simulink model "s9_template_2019a"  (R2019a)
settings: Solver=ode4  StartTime=0.0  StopTime=inf  FixedStep=P_sim_dt  RelTol=1e-3
InitFcn:
  | s6_data;
values from neighbouring files (symbols this model uses):
  init_psi = -pi/2    (= -1.57079632679)    [s6_data.m]
  init_s1 = a1boundary + P_width/2    (= 0.15)    [s6_data.m]
  init_s2 = a2total/2    (= 0.9)    [s6_data.m]
  P_delta_n_max = 1    [s6_data.m]
  P_delta_n_min = -1    [s6_data.m]
  P_dt = 20e-3    (= 0.02)    [s6_data.m]
  P_kr = 1/P_ku * sqrt((P_Ti^2*P_omega_d^2 + P_T^2*P_Ti^2*P_omega_d^4) /     (1 + P_Ti^2*P_omega_d^2))    [ex6_1.m]    (also in s6_data.m = sqrt((P_omega_d^2*P_T*P_Ti)^2 + (P_omega_d*P_Ti)^2) /      ()
  P_Ta = 0.02    [ex6_1.m]    (also in s6_data.m)
  P_Ti = (tan(P_phires_arc - pi + P_Tt*P_omega_d) * P_T * P_omega_d - 1)/     (P_T*P_omega_d^2 + tan(P_phires_arc - pi + P_Tt*P_omega_d) * P_omega_d )    [ex6_1.m]    (also in s6_data.m = tan(P_phi_res - pi/2 + P_omega_d*P_Tt + atan(P_omega_d*P_T)))
  P_Tw = 1000e-3    (= 1)    [ex6_1.m]    (also in s6_data.m = 0.3)
  P_un_max = 1    [s6_data.m]
  P_un_min = -1    [s6_data.m]
  P_v_fb_border = 0.1    [s6_data.m]
  P_vTarget = 0.3    [s6_data.m]
  P_w_breakslen = uint32(length(path.points))    [s6_data.m]
  P_w_coefs = zeros(SPLINE.Elements(3).Dimensions)    [s6_data.m]
  P_w_points = zeros(SPLINE.Elements(2).Dimensions)    [s6_data.m]
  P_w_segments = uint32(zeros(SPLINE.Elements(4).Dimensions))    [s6_data.m]
  track = mbc_track_display(track, 0.1, [ 0 a1total 0 a2total ])    [s6_data.m]
undefined symbols (not defined in the file or in its folder): CarInputsCmdForward, disableLaneMonitor, isnew, lapCount, ManeuverTypePathFollow, P_p_Bf, P_p_Br, P_p_Cf, P_p_Cr, P_p_delta_max, P_p_delta_min, P_p_Df, P_p_Dr, P_p_frontaxle_1, P_p_J, P_p_k, P_p_l, P_p_m, P_p_rearaxle_1, P_p_T, P_p_un_max, P_p_un_min, P_p_un_slow_max, P_p_un_slow_min, P_p_uTt, P_p_v_min, type, vmax, xManeuverEnd
libraries: mad_lib_template x1
settings Model: Creator=hmekiedj  LastModifiedBy=exdestruction
settings DataIOCC: ReturnWorkspaceOutputs=off
settings DebuggingCC: ArithmeticOperatorsInVariantConditions=warning
settings SFSimCC: SimUseLocalCustomCode=off
settings RTWCC: RTWUseLocalCustomCode=off

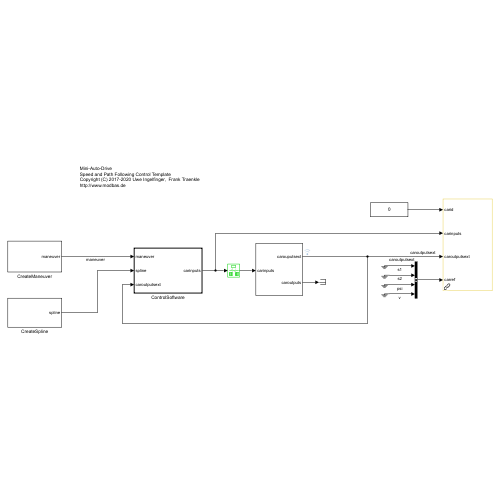
[thumbnail: Simulink's stored preview of the top-level diagram]
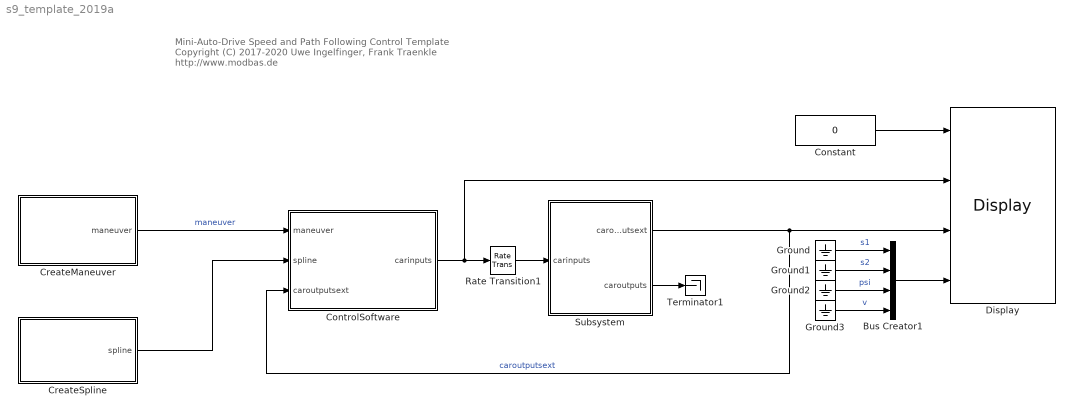
== system s9_template_2019a ==
  note: Mini-Auto-Drive
      | Speed and Path Following Control Template
      | Copyright (C) 2017-2020 Uwe Ingelfinger,  Frank Traenkle
      | http://www.modbas.de
  Bus Creator1 : BusCreator  Inputs=4
  Constant : Constant  Value=0
  ControlSoftware : Subsystem  TreatAsAtomicUnit=on  SystemSampleTime=P_dt
  CreateManeuver : Subsystem
  CreateSpline : Subsystem
  Display : mad_lib_template/Display  SystemSampleTime=-1  Latency=0  AutoFrameSizeCalculation=off
  Ground{,1..3} (4 alike) : Ground
  Rate Transition1 : RateTransition
  Subsystem : Subsystem
  Terminator1 : Terminator
  wires:
  Bus Creator1/1 -> Display/4
  Ground/1 -> Bus Creator1/1  "s1"
  Ground1/1 -> Bus Creator1/2  "s2"
  Ground2/1 -> Bus Creator1/3  "psi"
  Ground3/1 -> Bus Creator1/4  "v"
  Subsystem/1(carouputsext) -> ControlSoftware/3(caroutputsext), Display/3  "caroutputsext"
  Rate Transition1/1 -> Subsystem/1(carinputs)
  Constant/1 -> Display/1
  ControlSoftware/1(carinputs) -> Display/2, Rate Transition1/1
  CreateManeuver/1(maneuver) -> ControlSoftware/1(maneuver)  "maneuver"
  Subsystem/2(caroutputs) -> Terminator1/1
  CreateSpline/1(spline) -> ControlSoftware/2(spline)

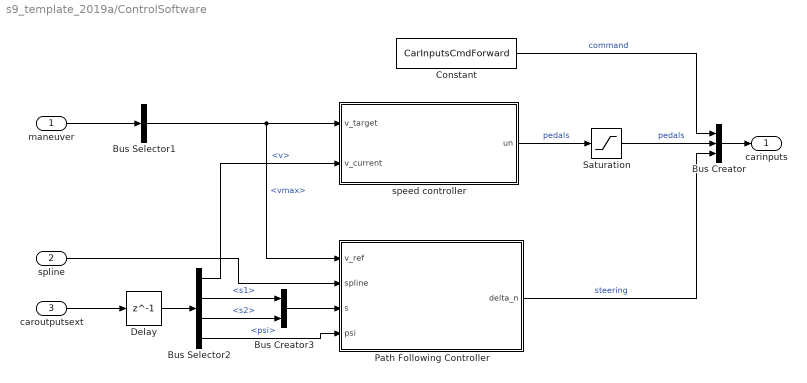
== system s9_template_2019a/ControlSoftware ==
  maneuver : Inport
  spline : Inport  Port=2
  caroutputsext : Inport  Port=3
  Bus Creator : BusCreator  Inputs=3
  Bus Creator3 : BusCreator  Inputs=2
  Bus Selector1 : BusSelector  OutputSignals=vmax
  Bus Selector2 : BusSelector  OutputSignals=v,s1,s2,psi
  Constant : Constant  Value=CarInputsCmdForward  SampleTime=-1
  Delay : Delay  DelayLength=1
  Path Following Controller : Subsystem
  Saturation : Saturate  UpperLimit=P_un_max  LowerLimit=P_un_min
  speed controller : Subsystem  TreatAsAtomicUnit=on  SystemSampleTime=P_dt
      settings: MinAlgLoopOccurrences=on
  carinputs : Outport
  wires:
  caroutputsext/1 -> Delay/1
  Bus Creator/1 -> carinputs/1
  maneuver/1 -> Bus Selector1/1
  speed controller/1(un) -> Saturation/1  "pedals"
  Saturation/1 -> Bus Creator/2  "pedals"
  Constant/1 -> Bus Creator/1  "command"
  Path Following Controller/1(delta_n) -> Bus Creator/3  "steering"
  Bus Creator3/1 -> Path Following Controller/3(s)
  Bus Selector2/1 -> speed controller/2(v_current)  "<v>"
  Bus Selector2/2 -> Bus Creator3/1  "<s1>"
  Bus Selector2/4 -> Path Following Controller/4(psi)  "<psi>"
  Bus Selector2/3 -> Bus Creator3/2  "<s2>"
  Bus Selector1/1 -> Path Following Controller/1(v_ref), speed controller/1(v_target)  "<vmax>"
  Delay/1 -> Bus Selector2/1
  spline/1 -> Path Following Controller/2(spline)

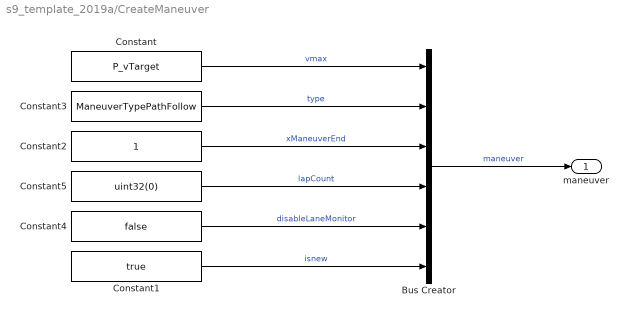
== system s9_template_2019a/CreateManeuver ==
  Bus Creator : BusCreator  Inputs=vmax,type,xManeuverEnd,lapCount,disableLaneMonitor,isnew  OutDataTypeStr=Bus: MANEUVER  NonVirtualBus=on
  Constant : Constant  Value=P_vTarget
  Constant1 : Constant  Value=true
  Constant2 : Constant
  Constant3 : Constant  Value=ManeuverTypePathFollow
  Constant4 : Constant  Value=false
  Constant5 : Constant  Value=uint32(0)
  maneuver : Outport
  wires:
  Bus Creator/1 -> maneuver/1  "maneuver"
  Constant3/1 -> Bus Creator/2  "type"
  Constant2/1 -> Bus Creator/3  "xManeuverEnd"
  Constant4/1 -> Bus Creator/5  "disableLaneMonitor"
  Constant5/1 -> Bus Creator/4  "lapCount"
  Constant1/1 -> Bus Creator/6  "isnew"
  Constant/1 -> Bus Creator/1  "vmax"

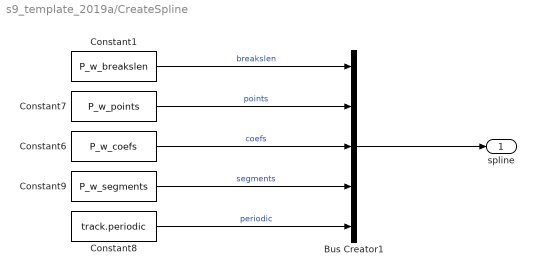
== system s9_template_2019a/CreateSpline ==
  Bus Creator1 : BusCreator  Inputs=5  OutDataTypeStr=Bus: SPLINE  NonVirtualBus=on
  Constant1 : Constant  Value=P_w_breakslen  VectorParams1D=off
  Constant6 : Constant  Value=P_w_coefs  VectorParams1D=off
  Constant7 : Constant  Value=P_w_points  VectorParams1D=off
  Constant8 : Constant  Value=track.periodic  VectorParams1D=off
  Constant9 : Constant  Value=P_w_segments  VectorParams1D=off
  spline : Outport
  wires:
  Constant1/1 -> Bus Creator1/1  "breakslen"
  Constant8/1 -> Bus Creator1/5  "periodic"
  Constant9/1 -> Bus Creator1/4  "segments"
  Constant6/1 -> Bus Creator1/3  "coefs"
  Constant7/1 -> Bus Creator1/2  "points"
  Bus Creator1/1 -> spline/1

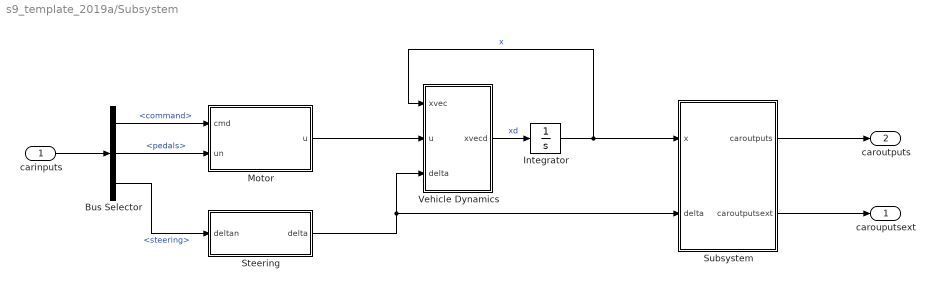
== system s9_template_2019a/Subsystem ==
  carinputs : Inport
  Bus Selector : BusSelector  OutputSignals=command,pedals,steering
  Integrator : Integrator  InitialCondition=[ 0; init_s1; init_s2; init_psi; 0; 0; 0]
  Motor : Subsystem
  Steering : Subsystem
  Subsystem : Subsystem
  Vehicle Dynamics : MATLAB Function  TreatAsAtomicUnit=on
  carouputsext : Outport
  caroutputs : Outport  Port=2
  wires:
  Vehicle Dynamics/1(xvecd) -> Integrator/1  "xd"
  Motor/1(u) -> Vehicle Dynamics/2(u)
  carinputs/1 -> Bus Selector/1
  Integrator/1 -> Subsystem/1(x), Vehicle Dynamics/1(xvec)  "x"
  Bus Selector/3 -> Steering/1(deltan)  "<steering>"
  Steering/1(delta) -> Subsystem/2(delta), Vehicle Dynamics/3(delta)
  Bus Selector/2 -> Motor/2(un)  "<pedals>"
  Bus Selector/1 -> Motor/1(cmd)  "<command>"
  Subsystem/1(caroutputs) -> caroutputs/1
  Subsystem/2(caroutputsext) -> carouputsext/1

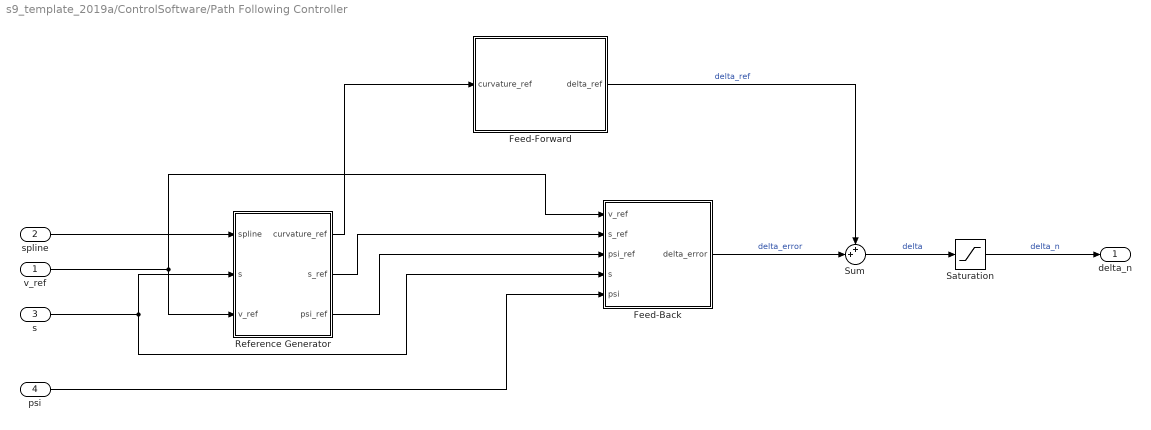
== system s9_template_2019a/ControlSoftware/Path Following Controller ==
  v_ref : Inport
  spline : Inport  Port=2
  s : Inport  Port=3
  psi : Inport  Port=4
  Feed-Back : Subsystem
  Feed-Forward : Subsystem
  Reference Generator : Subsystem
  Saturation : Saturate  UpperLimit=P_delta_n_max  LowerLimit=P_delta_n_min
  Sum : Sum  Inputs=++|
  delta_n : Outport
  wires:
  Saturation/1 -> delta_n/1  "delta_n"
  Sum/1 -> Saturation/1  "delta"
  Feed-Back/1(delta_error) -> Sum/2  "delta_error"
  Reference Generator/2(s_ref) -> Feed-Back/2(s_ref)
  Reference Generator/3(psi_ref) -> Feed-Back/3(psi_ref)
  s/1 -> Feed-Back/4(s), Reference Generator/2(s)
  psi/1 -> Feed-Back/5(psi)
  Reference Generator/1(curvature_ref) -> Feed-Forward/1(curvature_ref)
  v_ref/1 -> Feed-Back/1(v_ref), Reference Generator/3(v_ref)
  Feed-Forward/1(delta_ref) -> Sum/1  "delta_ref"
  spline/1 -> Reference Generator/1(spline)

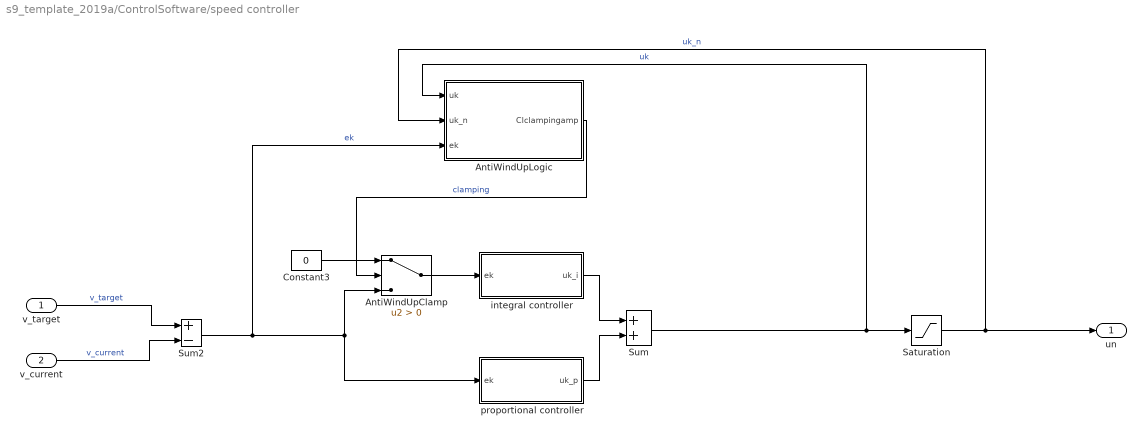
== system s9_template_2019a/ControlSoftware/speed controller ==
  v_target : Inport
  v_current : Inport  Port=2
  AntiWindUpClamp : Switch  Criteria=u2 > Threshold
  AntiWindUpLogic : Subsystem
  Constant3 : Constant  Value=0
  Saturation : Saturate  UpperLimit=P_un_max  LowerLimit=P_un_min
  Sum : Sum
  Sum2 : Sum  Inputs=+-
  integral controller : Subsystem
  proportional controller : Subsystem
  un : Outport
  wires:
  Saturation/1 -> AntiWindUpLogic/2(uk_n), un/1  "uk_n"
  Sum2/1 -> AntiWindUpLogic/3(ek), AntiWindUpClamp/3, proportional controller/1(ek)  "ek"
  Sum/1 -> Saturation/1, AntiWindUpLogic/1(uk)  "uk"
  v_target/1 -> Sum2/1  "v_target"
  v_current/1 -> Sum2/2  "v_current"
  Constant3/1 -> AntiWindUpClamp/1
  AntiWindUpLogic/1(Clclampingamp) -> AntiWindUpClamp/2  "clamping"
  proportional controller/1(uk_p) -> Sum/2
  integral controller/1(uk_i) -> Sum/1
  AntiWindUpClamp/1 -> integral controller/1(ek)

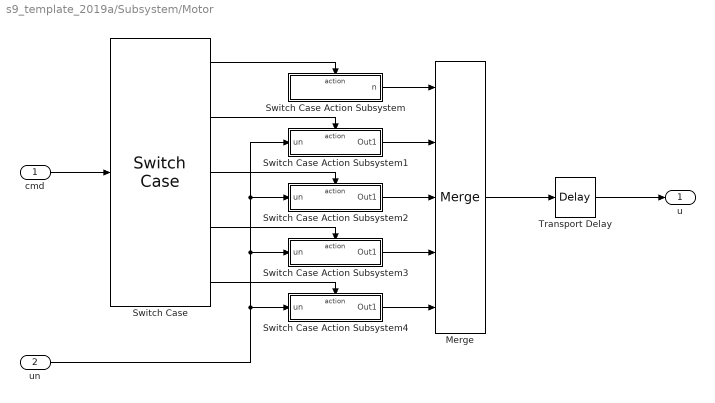
== system s9_template_2019a/Subsystem/Motor ==
  cmd : Inport
  un : Inport  Port=2
  Merge : Merge  Inputs=5
  Switch Case : SwitchCase  CaseConditions={0,1,2,3}
  Switch Case Action Subsystem : Subsystem  TreatAsAtomicUnit=on
  Switch Case Action Subsystem1 : Subsystem  TreatAsAtomicUnit=on
  Switch Case Action Subsystem2 : Subsystem  TreatAsAtomicUnit=on
  Switch Case Action Subsystem3 : Subsystem  TreatAsAtomicUnit=on
  Switch Case Action Subsystem4 : Subsystem  TreatAsAtomicUnit=on
  Transport Delay : TransportDelay  DelayTime=P_p_uTt
  u : Outport
  wires:
  cmd/1 -> Switch Case/1
  un/1 -> Switch Case Action Subsystem1/1(un), Switch Case Action Subsystem2/1(un), Switch Case Action Subsystem3/1(un), Switch Case Action Subsystem4/1(un)
  Switch Case Action Subsystem/1(n) -> Merge/1
  Switch Case Action Subsystem1/1(Out1) -> Merge/2
  Switch Case Action Subsystem2/1(Out1) -> Merge/3
  Switch Case Action Subsystem3/1(Out1) -> Merge/4
  Switch Case Action Subsystem4/1(Out1) -> Merge/5
  Merge/1 -> Transport Delay/1
  Transport Delay/1 -> u/1
  Switch Case/3 -> Switch Case Action Subsystem2/Action
  Switch Case/1 -> Switch Case Action Subsystem/Action
  Switch Case/2 -> Switch Case Action Subsystem1/Action
  Switch Case/4 -> Switch Case Action Subsystem3/Action
  Switch Case/5 -> Switch Case Action Subsystem4/Action

== system s9_template_2019a/Subsystem/Steering ==
  deltan : Inport
  Saturation : Saturate  UpperLimit=P_p_delta_max  LowerLimit=P_p_delta_min
  Transport Delay : TransportDelay  DelayTime=P_p_uTt
  delta : Outport
  wires:
  deltan/1 -> Saturation/1
  Saturation/1 -> Transport Delay/1
  Transport Delay/1 -> delta/1

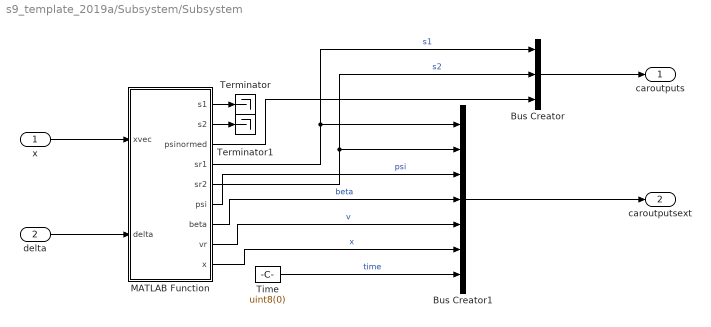
== system s9_template_2019a/Subsystem/Subsystem ==
  x : Inport
  delta : Inport  Port=2
  Bus Creator : BusCreator  Inputs=3
  Bus Creator1 : BusCreator  Inputs=7  OutDataTypeStr=Bus: CAROUTPUTSEXT  NonVirtualBus=on
  MATLAB Function : MATLAB Function  TreatAsAtomicUnit=on
  Terminator : Terminator
  Terminator1 : Terminator
  Time : Constant  Value=uint8(0)
  caroutputs : Outport
  caroutputsext : Outport  Port=2
  wires:
  MATLAB Function/8(vr) -> Bus Creator1/5  "v"
  MATLAB Function/6(psi) -> Bus Creator1/3  "psi"
  MATLAB Function/5(sr2) -> Bus Creator/2, Bus Creator1/2  "s2"
  MATLAB Function/7(beta) -> Bus Creator1/4  "beta"
  MATLAB Function/9(x) -> Bus Creator1/6  "x"
  Time/1 -> Bus Creator1/7  "time"
  MATLAB Function/4(sr1) -> Bus Creator/1, Bus Creator1/1  "s1"
  Bus Creator1/1 -> caroutputsext/1
  x/1 -> MATLAB Function/1(xvec)
  delta/1 -> MATLAB Function/2(delta)
  Bus Creator/1 -> caroutputs/1
  MATLAB Function/3(psinormed) -> Bus Creator/3
  MATLAB Function/1(s1) -> Terminator/1
  MATLAB Function/2(s2) -> Terminator1/1

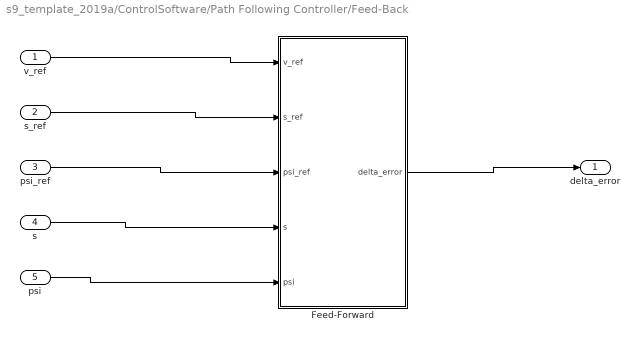
== system s9_template_2019a/ControlSoftware/Path Following Controller/Feed-Back ==
  v_ref : Inport
  s_ref : Inport  Port=2
  psi_ref : Inport  Port=3
  s : Inport  Port=4
  psi : Inport  Port=5
  Feed-Forward : MATLAB Function  TreatAsAtomicUnit=on
  delta_error : Outport
  wires:
  Feed-Forward/1(delta_error) -> delta_error/1
  v_ref/1 -> Feed-Forward/1(v_ref)
  s_ref/1 -> Feed-Forward/2(s_ref)
  psi_ref/1 -> Feed-Forward/3(psi_ref)
  s/1 -> Feed-Forward/4(s)
  psi/1 -> Feed-Forward/5(psi)

== system s9_template_2019a/ControlSoftware/Path Following Controller/Feed-Forward ==
  curvature_ref : Inport
  MATLAB Function : MATLAB Function  TreatAsAtomicUnit=on
  delta_ref : Outport
  wires:
  curvature_ref/1 -> MATLAB Function/1(curvature_ref)
  MATLAB Function/1(delta_ref) -> delta_ref/1

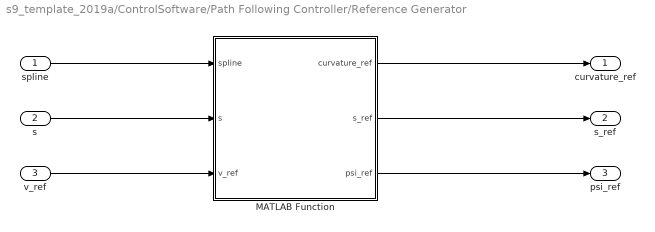
== system s9_template_2019a/ControlSoftware/Path Following Controller/Reference Generator ==
  spline : Inport
  s : Inport  Port=2
  v_ref : Inport  Port=3
  MATLAB Function : MATLAB Function  TreatAsAtomicUnit=on
  curvature_ref : Outport
  s_ref : Outport  Port=2
  psi_ref : Outport  Port=3
  wires:
  v_ref/1 -> MATLAB Function/3(v_ref)
  s/1 -> MATLAB Function/2(s)
  MATLAB Function/1(curvature_ref) -> curvature_ref/1
  MATLAB Function/2(s_ref) -> s_ref/1
  MATLAB Function/3(psi_ref) -> psi_ref/1
  spline/1 -> MATLAB Function/1(spline)

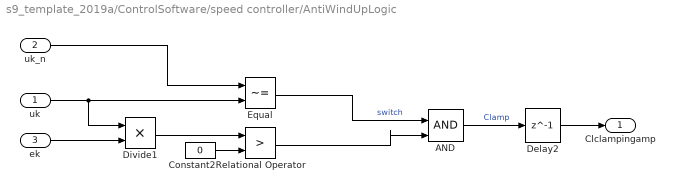
== system s9_template_2019a/ControlSoftware/speed controller/AntiWindUpLogic ==
  uk : Inport
  uk_n : Inport  Port=2
  ek : Inport  Port=3
  AND : Logic  IconShape=distinctive  AllPortsSameDT=off  OutDataTypeStr=boolean
  Constant2 : Constant  Value=0
  Delay2 : Delay  DelayLength=1  SampleTime=P_Ta
  Divide1 : Product  Inputs=**
  Equal : RelationalOperator  Operator=~=  OutDataTypeStr=boolean  RndMeth=Simplest
  Relational Operator : RelationalOperator  Operator=>  OutDataTypeStr=boolean  RndMeth=Simplest
  Clclampingamp : Outport
  wires:
  Constant2/1 -> Relational Operator/2
  Divide1/1 -> Relational Operator/1
  Relational Operator/1 -> AND/2
  Equal/1 -> AND/1  "switch"
  Delay2/1 -> Clclampingamp/1
  uk/1 -> Equal/2, Divide1/1
  ek/1 -> Divide1/2
  uk_n/1 -> Equal/1
  AND/1 -> Delay2/1  "Clamp"

== system s9_template_2019a/ControlSoftware/speed controller/integral controller ==
  ek : Inport
  Delay : Delay  DelayLength=1  SampleTime=P_Ta
  Gain : Gain  Gain=P_kr
  Gain1 : Gain  Gain=P_Ta
  Gain2 : Gain  Gain=1/P_Ti
  Sum1 : Sum
  uk_i : Outport
  wires:
  ek/1 -> Gain/1
  Sum1/1 -> uk_i/1, Delay/1
  Delay/1 -> Sum1/1
  Gain1/1 -> Gain2/1
  Gain/1 -> Gain1/1
  Gain2/1 -> Sum1/2

== system s9_template_2019a/ControlSoftware/speed controller/proportional controller ==
  ek : Inport
  ProportionalGain : Gain  Gain=P_kr
  uk_p : Outport
  wires:
  ek/1 -> ProportionalGain/1
  ProportionalGain/1 -> uk_p/1

== system s9_template_2019a/Subsystem/Motor/Switch Case Action Subsystem ==
  Action Port : ActionPort
  Constant : Constant  Value=0
  n : Outport
  wires:
  Constant/1 -> n/1

== system s9_template_2019a/Subsystem/Motor/Switch Case Action Subsystem1 ==
  un : Inport
  Action Port : ActionPort
  Saturation : Saturate  UpperLimit=P_p_un_max  LowerLimit=0
  Out1 : Outport
  wires:
  un/1 -> Saturation/1
  Saturation/1 -> Out1/1

== system s9_template_2019a/Subsystem/Motor/Switch Case Action Subsystem2 ==
  un : Inport
  Action Port : ActionPort
  Saturation : Saturate  UpperLimit=0  LowerLimit=P_p_un_min
  Out1 : Outport
  wires:
  un/1 -> Saturation/1
  Saturation/1 -> Out1/1

== system s9_template_2019a/Subsystem/Motor/Switch Case Action Subsystem3 ==
  un : Inport
  Action Port : ActionPort
  Saturation : Saturate  UpperLimit=P_p_un_slow_max  LowerLimit=P_p_un_slow_min
  Out1 : Outport
  wires:
  un/1 -> Saturation/1
  Saturation/1 -> Out1/1

== system s9_template_2019a/Subsystem/Motor/Switch Case Action Subsystem4 ==
  un : Inport
  Action Port : ActionPort
  Saturation : Saturate  UpperLimit=P_p_un_max  LowerLimit=P_p_un_min
  Out1 : Outport
  wires:
  un/1 -> Saturation/1
  Saturation/1 -> Out1/1

== matlab function s9_template_2019a/Subsystem/Subsystem/MATLAB Function ==
  data: s1 output; s2 output; xvec input; delta input; psinormed output; sr1 output; sr2 output; psi output; beta output; vr output; x output; P_p_rearaxle_1 parameter; P_p_v_min parameter; P_p_l parameter
function [s1, s2, psinormed, sr1, sr2, psi, beta, vr, x] = outputs(xvec, delta, P_p_rearaxle_1, P_p_v_min, P_p_l)

temp2 = zeros(1,4);
temp2 = xvec;
vc1 = temp2(1);
s1 = temp2(2);
s2 = temp2(3);
psi = temp2(4);
x = temp2(7);

psinormed = mod(psi, 2*pi);
if psinormed > pi
    psinormed = psinormed - 2*pi;
end
beta = 0;
sr1 = s1 - P_p_rearaxle_1 * cos(psi);
sr2 = s2 - P_p_rearaxle_1 * sin(psi);
vr = vc1;
end

== matlab function s9_template_2019a/Subsystem/Vehicle Dynamics ==
  data: xvec input; u input; delta input; xvecd output; P_p_Br parameter; P_p_Bf parameter; P_p_Cr parameter; P_p_Cf parameter; P_p_Dr parameter; P_p_Df parameter; P_p_rearaxle_1 parameter; P_p_frontaxle_1 parameter; P_p_m parameter; P_p_J parameter; P_p_k parameter; P_p_T parameter; P_p_v_min parameter; P_p_l parameter
function xvecd = dynamics(xvec, u, delta, P_p_Br, P_p_Bf, P_p_Cr, P_p_Cf, P_p_Dr, P_p_Df, ...
    P_p_rearaxle_1, P_p_frontaxle_1, P_p_m, P_p_J, P_p_k, P_p_T, P_p_v_min, P_p_l)

temp = zeros(7,1);
temp = xvec;

vc1 = temp(1);
psi = temp(4);
psid = temp(5);
vc2 = temp(6);

if abs(vc1) > P_p_v_min % avoid model singularity at zero speed
    %% bicycle model with Magic Tire
    spsi = sin(psi);
    cpsi = cos(psi);
    sdelta = sin(delta);
    cdelta = cos(delta);
    
    % wheel slip angles
    alphaf = -atan2(vc2 + P_p_frontaxle_1 * psid, vc1) + delta;
    alphar = -atan2(vc2 - P_p_rearaxle_1 * psid, vc1);
    % wheel forces
    Ff = P_p_Df * sin(P_p_Cf * atan(P_p_Bf * alphaf));
    Fr = P_p_Dr * sin(P_p_Cr * atan(P_p_Br * alphar));    
    % logitudinal dynamics (momentum balance)
    vc1d = (-Ff * sdelta + P_p_m * vc2 * psid) / P_p_m ...
            - vc1/P_p_T + P_p_k/P_p_T * u;
    % kinematics
    s1d = vc1 * cpsi - vc2 * spsi;
    s2d = vc1 * spsi + vc2 * cpsi;
    % rotational dynamics (moment of momentum balance)
    psidd = (Ff * P_p_frontaxle_1 * cdelta - Fr * P_p_rearaxle_1) / P_p_J;
    % lateral dynamics (momentum balance)
    vc2d = (Ff * cdelta + Fr - P_p_m * vc1 * psid)/P_p_m;
    % driven arc length of rear axle center
    xd = vc1;
else % near zero speed
    %% longitudinal dynamics of rear axle
    a = P_p_rearaxle_1;
    l = P_p_l;
    spsi = sin(psi);
    cpsi = cos(psi);
    tdelta = tan(delta);
    vc2 = a/l * vc1 * tdelta;
    vc1d = (-vc1 + P_p_k * u) / P_p_T; % -(a^2+P_p_J/P_p-m)/l^2*vc1*tdelta*deltad
    s1d = vc1 * cpsi - vc2 * spsi;
    s2d = vc1 * spsi + vc2 * cpsi;
    psid = vc1 / l * tdelta;
    psidd = 0; % vc1d / l * tdelta + vc1/l * deltad * (1 + tdelta*delta)
    vc2d = 0 ; % a * psidd;
    xd = vc1;
end
    
xvecd = [ vc1d; s1d; s2d; psid; psidd; vc2d; xd ];
end

== matlab function s9_template_2019a/ControlSoftware/Path Following Controller/Feed-Back/Feed-Forward ==
  data: v_ref input; delta_error output; s_ref input; psi_ref input; s input; psi input; P_p_l parameter; P_Tw parameter; P_v_fb_border parameter
function delta_error = feed_back(v_ref, s_ref, psi_ref, s, psi, P_p_l, P_Tw, P_v_fb_border)


if abs(v_ref) < P_v_fb_border
    v_ref = sign(v_ref) .* P_v_fb_border;
end

normal_vector_ref = [-sin(psi_ref); cos(psi_ref)];
psi_error = psi - psi_ref;
psi_error = mod(psi_error, 2*pi);
if psi_error > pi
    psi_error = psi_error - 2*pi;
end
s_c2e = (s - s_ref)' * normal_vector_ref;
delta_error = -(P_p_l*s_c2e)/(P_Tw * v_ref)^2 - (2*P_p_l*psi_error)/(P_Tw*v_ref);

== matlab function s9_template_2019a/ControlSoftware/Path Following Controller/Feed-Forward/MATLAB Function ==
  data: delta_ref output; curvature_ref input; P_p_l parameter
function delta_ref = feed_forward(curvature_ref, P_p_l)

delta_ref = atan(P_p_l * curvature_ref);

== matlab function s9_template_2019a/ControlSoftware/Path Following Controller/Reference Generator/MATLAB Function ==
  data: spline input; s input; v_ref input; curvature_ref output; s_ref output; psi_ref output; P_Tt parameter
function [curvature_ref, s_ref, psi_ref] = reference_generator(spline, s, v_ref, P_Tt)


[w, ~]  = mbc_spline_get_reference(s, spline.breakslen, spline.points, spline.coefs, spline.periodic, v_ref, P_Tt);

s_ref = [w(3); w(4)];
psi_ref = w(2);
curvature_ref = w(5);
